simulink model "busTest"  (R2015a)
settings: Solver=ode45  StartTime=0.0  StopTime=10.0  RelTol=1e-3
settings Model: Creator=John  LastModifiedBy=John

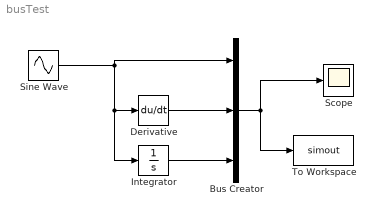
== system busTest ==
  Bus Creator : BusCreator  Inputs=3
  Derivative : Derivative
  Integrator : Integrator
  Scope : Scope
  Sine Wave : Sin  Frequency=20  SampleTime=0  VectorParams1D=off
  To Workspace : ToWorkspace  VariableName=simout  SaveFormat=Timeseries  SampleTime=-1
  wires:
  Sine Wave/1 -> Bus Creator/1, Integrator/1, Derivative/1
  Derivative/1 -> Bus Creator/2
  Bus Creator/1 -> Scope/1, To Workspace/1
  Integrator/1 -> Bus Creator/3
